simulink model "CapturePointAlgorithm"  (R2020a)
settings: Solver=VariableStepAuto  StartTime=0.0  StopTime=inf  RelTol=1e-3
values from neighbouring files (symbols this model uses):
  Ts = 0.005    [startupWalkingRobot.m]
undefined symbols (not defined in the file or in its folder): gcbh
settings Model: EnablePacing=on  Creator=brian  LastModifiedBy=brian

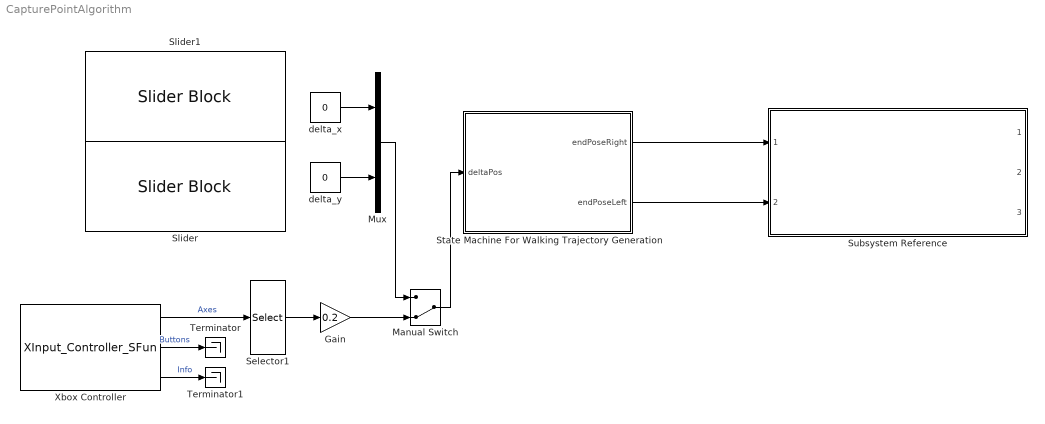
== system CapturePointAlgorithm ==
  Gain : Gain  Gain=0.2
  Manual Switch : ManualSwitch  CurrentSetting=0
  Mux : Mux  Inputs=2
  Selector1 : Selector  InputPortWidth=6  IndexOptions=Index vector (dialog)  Indices=[1 2]  OutputSizes=1
  Slider : SliderBlock  ScaleMin=-0.2  ScaleMax=0.2
  Slider1 : SliderBlock  ScaleMin=-0.2  ScaleMax=0.2
  State Machine For Walking Trajectory Generation : Stateflow chart  TreatAsAtomicUnit=on  SystemSampleTime=Ts
  Subsystem Reference : Subsystem  ReferencedSubsystem=WalkingRobotSubsystem
  Terminator : Terminator
  Terminator1 : Terminator
  Xbox Controller : S-Function  FunctionName=XInput_Controller_SFun  Parameters=1  SFunctionDeploymentMode=off  EnableBusSupport=off
  delta_x : Constant  StartFcn=set_param(gcbh,'Value','0')  Value=0
  delta_y : Constant  StartFcn=set_param(gcbh,'Value','0')  Value=0
  wires:
  Gain/1 -> Manual Switch/2
  Manual Switch/1 -> State Machine For Walking Trajectory Generation/1(deltaPos)
  Xbox Controller/1 -> Selector1/1  "Axes"
  Xbox Controller/3 -> Terminator1/1  "Info"
  Xbox Controller/2 -> Terminator/1  "Buttons"
  Mux/1 -> Manual Switch/1
  Selector1/1 -> Gain/1
  delta_y/1 -> Mux/2
  delta_x/1 -> Mux/1
  State Machine For Walking Trajectory Generation/2(endPoseLeft) -> Subsystem Reference/2
  State Machine For Walking Trajectory Generation/1(endPoseRight) -> Subsystem Reference/1

== stateflow chart CapturePointAlgorithm/State Machine For Walking Trajectory Generation ==
  state StandBy
    entry:
    idxmax = 0.5/TS;
    during:
    idx = idx + 1;
  note: Constants
      | Multiple Constants are used in this chart. Most constants are CAPITALIZED.
      | TS: sample time of trajectory
      | W: sqrt(g/zModel)
      | STEPTIME: duration of a single step
      | AD,BD, CD, DD: discrete state space representation of LIPM
      |
      | ZMODEL: the height of pendulum model; this is the height at which robot will walk
      | RHEIGHT: the height of the robot when standing straigh
      | RWDITH: the width of the robot
      |
      | TB_FR: the transform matrix from body to right foot at bend-knee position
      | TB_FL: the transfom matrix from body to left foot at bend-knee position
  note: Local Data
      | Multiple local variables are used in this chart. They are used in muliple area
      | Tworld_point : T generally refers to 4x4 transform matrix used to describe
      | position and oreintation of a body
      | Tw_sf : transform from world to swing foot
      | Tw_b : transform from world to 'capture-point body'
      | Tw_c : transform from world to actual body
      |
      | I created a transform for a imaginary body called 'capture-point body'. This
      | is just a state I keep track of user input. If the input was to move forward 0.1m
      | and to the right 0.2m, I move the 'capture-point body' by that amount. And
      | then based on that body, I get the necessary points (desired capture points).
  state BendKnee
    entry:
    endPoseRight =           [0 -1 0 RWIDTH/2;0 0 1 0;-1 0 0 -RHEIGHT;0 0 0 1];
    endPoseRightTarget = TB_FR;
    endPoseLeft =          [0 -1 0 -RWIDTH/2;0 0 1 0;-1 0 0 -RHEIGHT;0 0 0 1];
    endPoseLeftTarget = TB_FL;
    tduration = 2.0;
    xyzqtrajr = getTrajectory(endPoseRight, endPoseRightTarget, tduration);
    xyzqtrajl = getTrajectory(endPoseLeft, endPoseLeftTarget, tduration);
    idx = 1; idxmax = round(tduration/TS);
    endPoseRight = vec2Tform(xyzqtrajr(:,idx));
    endPoseLeft = vec2Tform(xyzqtrajl(:,idx));
    idx = idx + 1;
    during:
    endPoseRight = vec2Tform(xyzqtrajr(:,idx));
    endPoseLeft = vec2Tform(xyzqtrajl(:,idx));
    idx = idx + 1;
  state RightStance
    entry:
    getWalkingTrajectory(RIGHTSTANCE);
    during:
    endPoseRight = getStanceTform(RIGHTSTANCE);
    endPoseLeft = xyzq2Tform(swingXyzq(:,idx));
    idx = idx + 1;
  state LeftStance
    entry:
    getWalkingTrajectory(LEFTSTANCE);
    during:
    endPoseLeft = getStanceTform(LEFTSTANCE);
    endPoseRight = xyzq2Tform(swingXyzq(:,idx));
    idx = idx + 1;
  state WalkReady
    entry:
    endPoseRight = endPoseRightTarget;
    endPoseLeft = endPoseLeftTarget;
    endPoseRightTarget(1:3,4) = [0.0; 0.0; -ZMODEL];
    endPoseLeftTarget(1:3,4) = [-0.24; 0.0; -ZMODEL];
    tduration = 2.0;
    xyzqtrajr = getTrajectory(endPoseRight, endPoseRightTarget, tduration);
    xyzqtrajl = getTrajectory(endPoseLeft, endPoseLeftTarget, tduration);
    idxmax = round(tduration/TS);
    endPoseRight = vec2Tform(xyzqtrajr(:,idx));
    endPoseLeft = vec2Tform(xyzqtrajl(:,idx));
    idx = idx + 1;
    during:
    endPoseRight = vec2Tform(xyzqtrajr(:,idx));
    endPoseLeft = vec2Tform(xyzqtrajl(:,idx));
    idx = idx + 1;
  (default) -> StandBy : {idx = 1;}
  StandBy -> BendKnee : [idx > idxmax]
      | {idx = 1;}
  RightStance -> LeftStance : [idx > idxmax]{idx = 1;}
  BendKnee -> WalkReady : [idx > idxmax]
      | {idx = 1;}
  LeftStance -> RightStance : [idx > idxmax]{idx = 1;}
  WalkReady -> RightStance : [idx > idxmax]
      | {idx = 1;}
  data: rightStance function_input; whichStance function_input; tForm function_output; currMat function_input; targetMat function_input; taction function_input; xyzqtrajectory function_output; xyzqtrajectory function_output; currMat function_input; targetMat function_input; TS constant double =Ts; ZMODEL constant double =zModel; RWIDTH constant double =torso_width; RHEIGHT constant double =init_height; endPoseLeftTarget local size=[4,4]; endPoseRightTarget local size=[4,4]; endPoseRight output size=[4,4] =[0 -1 0 0.12;0 0 1 0;-1 0 0 -0.78;0 0 0 1]; endPoseLeft output size=[4,4] =[0 -1 0 -0.12;0 0 1 0;-1 0 0 -0.78;0 0 0 1]; xyzqtrajr local size=[7, 2500]; xyzqtrajl local size=[7, 2500]; tduration local; idxmax local; idx local; RIGHTSTANCE constant double =true; LEFTSTANCE constant double =false; deltaPos input size=2; TB_FR constant double size=[4,4] =[0 -1 0 torso_width/2;0 0 1 0;-1 0 0 -zModel;0 0 0 1];; TB_FL constant double size=[4,4] =[0 -1 0 -torso_width/2;0 0 1 0;-1 0 0 -zModel;0 0 0 1];; W constant double =w; STEPTIME constant double =desiredStepTime; Tw_b local =[1 0 0 0;0 1 0 0;0 0 1 zModel;0 0 0 1]; AD constant double size=[4, 4] =Ad; BD constant double size=[4,2] =Bd; CD constant double size=[2,4] =Cd; DD constant double size=[2,2] =Dd; state0 local =[x0 dx0 y0 dy0]'; state1 local =zeros(4,1); meas1 local =zeros(2,1); u0 local =zeros(2,1); SWINGHEIGHT constant double =0.1; measurementvec local =zeros(3,250); Tw_c local =[1 0 0 0;0 1 0 0;0 0 1 0;0 0 0 1]; Tw_c1 local =[1 0 0 0;0 1 0 0;0 0 1 0;0 0 0 1]; swingXyzq local size=[7,2500]; px local =0; py local =0; cx local =0; cy local =0
  function getWalkingTrajectory(rightStance):
    | function getWalkingTrajectory(rightStance)
    | % Tb, Tb1: The "capture-point body pose" is an capture-point body pose I keep track of to determine
    | % capture point. This is not really where the actual body of the robot will
    | % be, rather this is some pose that the robot will be around at during the middle
    | % of its stance trajectory. capture-point body pose is essentially something that helps
    | % me get the desired end-of-step capture point based on input. Remember the
    | % key input for this algorithm is the capture point. In the end I just want
    | % some capture point to work with. This capture-point body pose keep track of
    | % the input to give me that capture point. 
    | % The actual body of the robot is described with c Tc, Tw_c (center of
    | % body)
    | 
    | % transform from current capture-point body pose to next end of step capture-point 
    | % body pose
    | Tb_b1 = eye(4); 
    | Tb_b1(1,1) =  cos(0); Tb_b1(1,2) = sin(0);
    | Tb_b1(2,1) = -sin(0); Tb_b1(2,2) = cos(0);
    | Tb_b1(1,4) = deltaPos(1); 
    | Tb_b1(2,4) = deltaPos(2); 
    | 
    | % transform from body to foot's default (standing) pose
    | if rightStance % right stance 
    |     Tf = TB_FR; 
    |     Tstance = TB_FR; 
    |     Tswing  = TB_FL; 
    | else % left stance 
    |     Tf = TB_FL;  
    |     Tstance = TB_FL; 
    |     Tswing = TB_FR; 
    | end
    | 
    | % Tw_b:   transform from world to capture-point body 
    | % Tw_b1:  transform from world to capture-point body at end of step
    | % Tw_sf : transform from world to swing foot at beginning of step 
    | % Tw_sf1: transform from world to swing foot at end of step 
    | %         this is the next step's plant foot 
    | %         this is where the swing foot should land on 
    | %         this is based on desired capture point (thus input) 
    | Tw_b1  = Tw_b  * Tb_b1;
    | Tw_sf1 = Tw_b1 * Tswing;
    | 
    | % based on current capture point cx, cy and desired capture point (c-eos) 
    | % (which is where you will put your next stance foot down) at the
    | % end of step (cxeos, cyeos), calculate the pendulum base (ZMP) px and py. 
    | cxeos = Tw_sf1(1,4);
    | cyeos = Tw_sf1(2,4);
    | cx = state0(1) + state0(2)/W; % current capture point x
    | cy = state0(3) + state0(4)/W; % current capture point y 
    | px = findZMP(W, STEPTIME, cxeos, cx); 
    | py = findZMP(W, STEPTIME, cyeos, cy); 
    | u0 = [px; py];
    | 
    | % simulate the pendulum to get the trajectory out of it; 
    | % the ZMP (px, py) is the base of pendulum 
    | % This calculates the trajectory of robot's ACTUAL body w.r.t. world. 
    | % Tw_c  : transform from world to actual body at beginning of step 
    | % Tw_c1 : transform from world to actual body at end of step 
    | idxmax = round(STEPTIME/TS); 
    | simulateLipm();
    | Tw_c(1:3,4) = measurementvec(1:3,1);
    | Tw_c1(1:3,4) = measurementvec(1:3,idxmax); 
    | Tw_c1(1:3,1:3) = Tw_b1(1:3,1:3);
    | 
    | % Get the swing foot based on Tw_c
    | % swing foot beginning is basically where the plant(stance) foot was at the
    | % end of last step
    | if rightStance % right stance
    |     Tc_sf = endPoseLeft;
    | else % left stance
    |     Tc_sf = endPoseRight;
    | end 
    | Tc1_sf1 = TransformInverse(Tw_c1) * Tw_sf1;
    | 
    | % get the swing foot trajectory 
    | swingXyzq = generateSwingTraj(Tc_sf, Tc1_sf1);
    | end
  function tForm = getStanceTform(whichStance):
    | function tForm = getStanceTform(whichStance)
    | % Given COM trajectory w.r.t. world and ZMP, get the Tform of foot w.r.t.
    | % body at the idx 
    | Tw_b = eye(4,4); 
    | Tw_b(1:3,4) = measurementvec(1:3,idx); 
    | 
    | Tw_f = zeros(4,4); 
    | Tw_f(4,4) = 1; 
    | if whichStance == 1 % Right stance 
    |     Tw_f(1:3,1:3) = TB_FR(1:3,1:3); 
    | else % Left stance 
    |     Tw_f(1:3,1:3) = TB_FL(1:3,1:3);
    | end 
    | Tw_f(1:2,4) = [cx; cy];
    | 
    | Tb_w = TransformInverse(Tw_b); 
    | Tb_f = Tb_w * Tw_f;
    | 
    | tForm = Tb_f; 
    | end
  function simulateLipm:
    | function simulateLipm
    | % remember that in Stateflow, all variables are pretty much global
    | % variables
    |     measurementvec(3,:) = ZMODEL; 
    |     
    |     meas1 = CD*state0 + DD*u0;
    |     measurementvec(1:2,1) = meas1;
    |     for temp = 2:idxmax 
    |         state1 = AD*state0 + BD*u0;
    |         meas1  = CD*state1 + DD*u0;
    |         measurementvec(1:2,temp) = meas1;
    |         state0 = state1;
    |     end
    | end
  function xyzqtrajectory = getTrajectory(currMat, targetMat, taction):
    | function xyzqtrajectory = getTrajectory(currMat, targetMat, taction)
    | 
    | quat = quaternion(currMat(1:3,1:3), 'rotmat', 'frame'); 
    | quat = quat.compact; 
    | quattarget = quaternion(targetMat(1:3,1:3), 'rotmat', 'frame');
    | quattarget = quattarget.compact; 
    | 
    | x = currMat(1,4); y = currMat(2,4); z = currMat(3,4); 
    | xt = targetMat(1,4); yt = targetMat(2,4); zt = targetMat(3,4); 
    | 
    | currPts = [x y z quat]';
    | targetPts = [xt yt zt quattarget]'; 
    | 
    | wpts = [currPts targetPts]; 
    | tpts = [0 taction];
    | tvec = 0:TS:taction; 
    | 
    | [xyzqtrajectory, ~, ~, ~] = cubicpolytraj(wpts, tpts, tvec);
  function xyzqtrajectory = generateSwingTraj(currMat, targetMat):
    | function xyzqtrajectory = generateSwingTraj(currMat, targetMat)
    | 
    | quat = quaternion(currMat(1:3,1:3), 'rotmat', 'frame'); 
    | quat = quat.compact; 
    | quattarget = quaternion(targetMat(1:3,1:3), 'rotmat', 'frame');
    | quattarget = quattarget.compact; 
    | 
    | x0 = currMat(1,4);     y0 = currMat(2,4);     z0 = currMat(3,4); 
    | x2 = targetMat(1,4);   y2 = targetMat(2,4);   z2 = targetMat(3,4); 
    | x1 = (x0 + x2)/2;      y1 = (y0 + y2)/2;      z1 = z0 + SWINGHEIGHT; 
    | 
    | pts0 = [x0 y0 z0 quat]';
    | pts1 = [x1 y1 z1 quattarget]'; 
    | pts2 = [x2 y2 z2 quattarget]'; 
    | 
    | wpts = [pts0 pts1 pts2]; 
    | tpts = [0 STEPTIME/2 STEPTIME];
    | tvec = 0:TS:STEPTIME; 
    | 
    | [xyzqtrajectory, ~, ~, ~] = cubicpolytraj(wpts, tpts, tvec); 
    | end
